simulink model "AR4_robotv5"  (R2021a)
settings: Solver=VariableStepAuto  StartTime=0.0  StopTime=13.7896  RelTol=1e-3
undefined symbols (not defined in the file or in its folder): B, Levenberg, Marquardt, sigbuilder_block, Spline, X, Y, Z
libraries: sm_lib x612, nesl_utility x123, robotcorelib x28, simulink_extras x19, simulink x17, robotmaniplib x9
(part 1 of 14)
settings Model: PacingRate=0.350000  Creator=sense  LastModifiedBy=sense

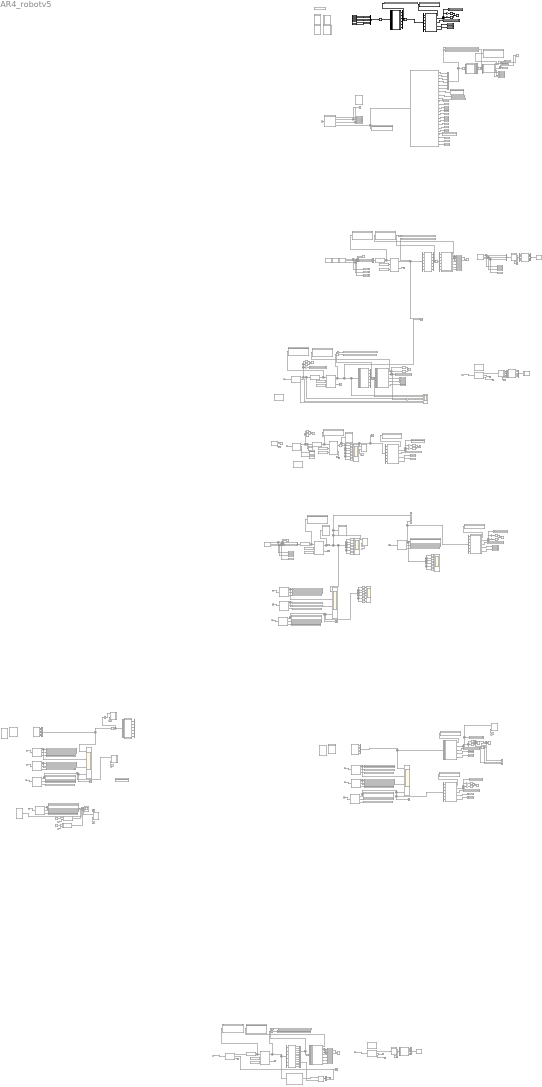
== system AR4_robotv5 ==
  note: task space
  note: joint space
  note: inverse kinematic
  note: Joint angles that achieve the given pose
  note: (Position vector)
  note: Controls importance of position/orientation
  note: Converts the 3D position (translation vector of end-effector) into a 4×4 homogeneous transformation matrix .
  note: Solves the inverse kinematics problem: Given a desired pose (position + orientation), compute the corresponding joint angles.
  note: take the waypoints of the trajectory
      | exert the angles + velocity + acceleration vectors
  note: (velocity vector)
  note: (accel vector)
  note: Joint angles that achieve the given pose
  note: (Position vector)
  note: Controls importance of position/orientation
  note: Converts the 3D position (translation vector of end-effector) into a 4×4 homogeneous transformation matrix .
  note: Solves the inverse kinematics problem: Given a desired pose (position + orientation), compute the corresponding joint angles.
  note: take the waypoints of the trajectory
      | exert the angles + velocity + acceleration vectors
  note: (velocity vector)
  note: (accel vector)
  note: joint space
  note: task space
  note: joint space
  Clock{,1..24} (25 alike) : Clock  Commented=on
  Constant{,2,4..5,8} (5 alike) : Constant  Commented=on  Value=[0 0 0 1 1 1]
  Constant{1,3,6..7,9} (5 alike) : Constant  Commented=on  Value=[0 0 0 0 0 0]
  Constant10 : Constant  Commented=on  Value=[140 60 -60 130 0 120]  VectorParams1D=off
  Constant11 : Constant  Commented=on  Value=[0 30 60 90 120 150 170 140]
  Constant12 : Constant  Commented=on  Value=[0 30 60 90 120 150 170 140]
  Coordinate Transformation Conversion{,1..4} (5 alike) : robotcorelib/Coordinate Transformation Conversion  Commented=on  InputRepresentation=Translation Vector  InputEulerSequence=ZYX  ShowTrVecInputPort=on  OutputRepresentation=Homogeneous Transformation  OutputEulerSequence=ZYX  ShowTrVecOutputPort=on  SimulateUsing=Interpreted execution
      settings: SourceProductBaseCode=NV,RO,RR,UV
  Degrees to Radians : simulink_extras/Transformations/Degrees to Radians  Commented=on
  Degrees to Radians1 : simulink_extras/Transformations/Degrees to Radians
  Degrees to Radians2 : simulink_extras/Transformations/Degrees to Radians  Commented=on
  Demux{,1..12,14,17..18} (16 alike) : Demux  Commented=on  Outputs=6
  Demux13 : Demux  Commented=on  Outputs=2
  Demux15 : Demux  Outputs=6
  Demux16 : Demux  Outputs=6
  Display{,1..76,82..83,85..109,191,263,267,302..304,306..307,309..323,331..332,360} (130 alike) : Display  Commented=on
      Display100 settings: Format=bank
      Display101 settings: Format=bank
      Display102 settings: Format=bank
      Display103 settings: Format=bank
      Display104 settings: Format=bank
      Display105 settings: Format=bank
      Display107 settings: Format=bank
      Display108 settings: Format=bank
      Display109 settings: Format=bank
      Display11 settings: Format=bank
      Display13 settings: Format=bank
      Display18 settings: Format=bank
      Display20 settings: Format=bank
      Display21 settings: Format=bank
      Display22 settings: Format=bank
      Display23 settings: Format=bank
      Display26 settings: Format=bank
      Display28 settings: Format=bank
      Display30 settings: Format=bank
      Display309 settings: Format=bank
      Display31 settings: Format=bank
      Display316 settings: Format=bank
      Display32 settings: Format=bank
      Display33 settings: Format=bank
      Display332 settings: Format=bank
      Display34 settings: Format=bank
      Display39 settings: Format=bank
      Display41 settings: Format=bank
      Display42 settings: Format=bank
      Display47 settings: Format=bank
      Display48 settings: Format=bank
      Display49 settings: Format=bank
      Display50 settings: Format=bank
      Display51 settings: Format=bank
      Display52 settings: Format=bank
      Display53 settings: Format=bank
      Display54 settings: Format=bank
      Display55 settings: Format=bank
      Display56 settings: Format=bank
      Display60 settings: Format=bank
      Display63 settings: Format=bank
      Display66 settings: Format=bank
      Display69 settings: Format=bank
      Display74 settings: Format=bank
      Display82 settings: Format=bank
      Display83 settings: Format=bank
      Display87 settings: Format=bank
      Display90 settings: Format=bank
      Display91 settings: Format=bank
      Display92 settings: Format=bank
      Display93 settings: Format=bank
      Display94 settings: Format=bank
      Display95 settings: Format=bank
      Display96 settings: Format=bank
      Display97 settings: Format=bank
      Display98 settings: Format=bank
      Display99 settings: Format=bank
  Display{77..81,84} (6 alike) : Display
      Display79 settings: Format=bank
  FIK13 : MATLAB Function  Commented=on  TreatAsAtomicUnit=on
  From Workspace : FromWorkspace  VariableName=q1
  From Workspace1 : FromWorkspace  VariableName=q2
  From Workspace2 : FromWorkspace  VariableName=q3
  From Workspace3 : FromWorkspace  VariableName=q4
  From Workspace4 : FromWorkspace  VariableName=q5
  From Workspace5 : FromWorkspace  VariableName=q6
  Gain : Gain  Commented=on  Gain=1000
  Gain{1..5,8..9} (7 alike) : Gain  Commented=on  Gain=0.001
  Gain6 : Gain  Gain=0.001
  Gain7 : Gain  Gain=0.001
  Get Jacobian : robotmaniplib/Get Jacobian  Commented=on  RigidBodyTree=robot  EndEffector=link7  SimulateUsing=Interpreted execution
      settings: SourceProductBaseCode=RO
  Inverse Kinematics{,1,3..4} (4 alike) : robotmaniplib/Inverse Kinematics  Commented=on  RigidBodyTree=robot  EndEffector=link7  ShowInfo=on  SolverName=Levenberg-Marquardt  EnforceJointLimits=on  MaxIterations=1500  MaxTime=10  GradientTolerance=1e-3  SolutionTolerance=1e-3  StepTolerance=1e-14  ErrorChangeTolerance=1e-3  UseErrorDamping=on  DampingBias=0.0025  SimulateUsing=Interpreted execution
  Inverse Kinematics2 : robotmaniplib/Inverse Kinematics  Commented=on  RigidBodyTree=robot  EndEffector=link7  ShowInfo=on  SolverName=Levenberg-Marquardt  EnforceJointLimits=on  MaxIterations=1500  MaxTime=10  GradientTolerance=1e-10  SolutionTolerance=1e-10  StepTolerance=1e-10  ErrorChangeTolerance=1e-10  UseErrorDamping=on  DampingBias=0.0025  SimulateUsing=Interpreted execution
  MATLAB Function : MATLAB Function  Commented=on  TreatAsAtomicUnit=on
  MATLAB Function1 : MATLAB Function  Commented=on  TreatAsAtomicUnit=on
  MATLAB Function10 : MATLAB Function  TreatAsAtomicUnit=on
  MATLAB Function11 : MATLAB Function  Commented=on  TreatAsAtomicUnit=on
  MATLAB Function12 : MATLAB Function  Commented=on  TreatAsAtomicUnit=on
  MATLAB Function13 : MATLAB Function  Commented=on  TreatAsAtomicUnit=on
  MATLAB Function14 : MATLAB Function  Commented=on  TreatAsAtomicUnit=on
  MATLAB Function15 : MATLAB Function  Commented=on  TreatAsAtomicUnit=on
  MATLAB Function16 : MATLAB Function  Commented=on  TreatAsAtomicUnit=on
  MATLAB Function17 : MATLAB Function  Commented=on  TreatAsAtomicUnit=on
  MATLAB Function2 : MATLAB Function  Commented=on  TreatAsAtomicUnit=on
  MATLAB Function3 : MATLAB Function  Commented=on  TreatAsAtomicUnit=on
  MATLAB Function4 : MATLAB Function  Commented=on  TreatAsAtomicUnit=on
  MATLAB Function5 : MATLAB Function  Commented=on  TreatAsAtomicUnit=on
  MATLAB Function6 : MATLAB Function  Commented=on  TreatAsAtomicUnit=on
  MATLAB Function7 : MATLAB Function  Commented=on  TreatAsAtomicUnit=on
  MATLAB Function8 : MATLAB Function  Commented=on  TreatAsAtomicUnit=on
  MATLAB Function9 : MATLAB Function  Commented=on  TreatAsAtomicUnit=on
  Matrix Multiply : Product  Commented=on  Multiplication=Matrix(*)
  Mux{,1,3..6,8..10,12,15,18} (12 alike) : Mux  Commented=on  Inputs=6
  Mux11 : Mux  Commented=on  Inputs=3
  Mux13 : Mux  Inputs=6
  Mux14 : Mux  Inputs=6
  Mux2 : Mux  Commented=on  Inputs=3
  Mux7 : Mux  Commented=on  Inputs=3
  Polynomial Trajectory : robotcorelib/Polynomial Trajectory  Commented=on  WaypointSource=Internal  Waypoints=|  TimePoints=[ 1, 2, 3, 4, 5 ]  TimeInterval=[ 1, 5 ]  Method=B-Spline  ParameterSource=Internal  VelocityBoundaryCondition=zeros(3, 5)  AccelerationBoundaryCondition=zeros(3, 5)  SimulateUsing=Interpreted execution
      | [0.3741, 0.5741, 0.5741, 0.3741, 0.3741;
      |  0.0000, 0.0000, 0.2000, 0.2000, 0.0000;
      |  0.4563, 0.4563, 0.4563, 0.4563, 0.4563]
  Polynomial Trajectory1 : robotcorelib/Polynomial Trajectory  Commented=on  WaypointSource=Internal  Waypoints=|  TimePoints=[ 1, 2, 3, 4, 5 ]  TimeInterval=[ 1, 5 ]  Method=B-Spline  ParameterSource=Internal  VelocityBoundaryCondition=zeros(3, 5)  AccelerationBoundaryCondition=zeros(3, 5)  SimulateUsing=Interpreted execution
      | [0.3741, 0.5741, 0.5741, 0.3741, 0.3741;
      |  0.0000, 0.0000, 0.2000, 0.2000, 0.0000;
      |  0.4563, 0.4563, 0.4563, 0.4563, 0.4563]
  Polynomial Trajectory10 : robotcorelib/Polynomial Trajectory  Commented=on  WaypointSource=Internal  Waypoints=thetatra  TimePoints=t  TimeInterval=time  Method=Cubic Polynomial  ParameterSource=Internal  VelocityBoundaryCondition=zeros(6,145)  AccelerationBoundaryCondition=zeros(6, 4);  SimulateUsing=Interpreted execution
  Polynomial Trajectory11 : robotcorelib/Polynomial Trajectory  Commented=on  WaypointSource=Internal  Waypoints=joint_angles_deg  TimePoints=[ 1, 2, 3, 4, 5 ]  TimeInterval=[0 1 2 3 4 5 6 7]  Method=B-Spline  ParameterSource=Internal  VelocityBoundaryCondition=zeros(3, 5)  AccelerationBoundaryCondition=zeros(3, 5)  SimulateUsing=Interpreted execution
  Polynomial Trajectory12 : robotcorelib/Polynomial Trajectory  Commented=on  WaypointSource=Internal  Waypoints=joint_angles_deg  TimePoints=[0 1 2 3 4 5 6 7 ]  TimeInterval=time  Method=Quintic Polynomial  ParameterSource=Internal  VelocityBoundaryCondition=zeros(6,8)  AccelerationBoundaryCondition=zeros(6,8)  SimulateUsing=Interpreted execution
  Polynomial Trajectory13 : robotcorelib/Polynomial Trajectory  Commented=on  WaypointSource=Internal  Waypoints=joint_angles_deg  TimePoints=[0 1 2 3 4 5 6 7]  TimeInterval=time  Method=Cubic Polynomial  ParameterSource=Internal  VelocityBoundaryCondition=zeros(6,8)  AccelerationBoundaryCondition=zeros(6, 4);  SimulateUsing=Interpreted execution
  Polynomial Trajectory14 : robotcorelib/Polynomial Trajectory  Commented=on  WaypointSource=Internal  Waypoints=joint_angles_deg  TimePoints=[ 1, 2, 3, 4, 5 ]  TimeInterval=[0 1 2 3 4 5 6 7]  Method=B-Spline  ParameterSource=Internal  VelocityBoundaryCondition=zeros(3, 5)  AccelerationBoundaryCondition=zeros(3, 5)  SimulateUsing=Interpreted execution
  Polynomial Trajectory15 : robotcorelib/Polynomial Trajectory  Commented=on  WaypointSource=Internal  Waypoints=joint1_angles  TimePoints=[ 1, 2, 3, 4, 5 ]  TimeInterval=[0 1 2 3 4 5 6 7]  Method=B-Spline  ParameterSource=Internal  VelocityBoundaryCondition=zeros(3, 5)  AccelerationBoundaryCondition=zeros(3, 5)  SimulateUsing=Interpreted execution
  Polynomial Trajectory2 : robotcorelib/Polynomial Trajectory  Commented=on  WaypointSource=Internal  Waypoints=|  TimePoints=[ 2, 4, 6, 8, 10 ]  TimeInterval=[ 1, 20 ]  Method=Quintic Polynomial  ParameterSource=Internal  VelocityBoundaryCondition=zeros(3, 5)  AccelerationBoundaryCondition=zeros(3, 5)  SimulateUsing=Interpreted execution
      | [0.3741, 0.5741, 0.5741, 0.3741, 0.3741;
      |  0.0000, 0.0000, 0.2000, 0.2000, 0.0000;
      |  0.4563, 0.4563, 0.4563, 0.4563, 0.4563]
  Polynomial Trajectory3 : robotcorelib/Polynomial Trajectory  Commented=on  WaypointSource=Internal  Waypoints=|  TimePoints=[ 2, 4, 6, 8, 10 ]  TimeInterval=[ 1, 20 ]  Method=Quintic Polynomial  ParameterSource=Internal  VelocityBoundaryCondition=zeros(3, 5)  AccelerationBoundaryCondition=zeros(3, 5)  SimulateUsing=Interpreted execution
      | [0.3741, 0.5741, 0.5741, 0.3741, 0.3741;
      |  0.0000, 0.0000, 0.2000, 0.2000, 0.0000;
      |  0.4563, 0.4563, 0.4563, 0.4563, 0.4563]
  Polynomial Trajectory4 : robotcorelib/Polynomial Trajectory  Commented=on  WaypointSource=Internal  Waypoints=joint_angles_deg  TimePoints=[ 1, 2, 3, 4, 5 ]  TimeInterval=[0 1 2 3 4 5 6 7]  Method=B-Spline  ParameterSource=Internal  VelocityBoundaryCondition=zeros(3, 5)  AccelerationBoundaryCondition=zeros(3, 5)  SimulateUsing=Interpreted execution
  Polynomial Trajectory5 : robotcorelib/Polynomial Trajectory  Commented=on  WaypointSource=Internal  Waypoints=joint_angles_deg  TimePoints=[0 1 2 3 4 5 6 7 ]  TimeInterval=time  Method=Quintic Polynomial  ParameterSource=Internal  VelocityBoundaryCondition=zeros(6,8)  AccelerationBoundaryCondition=zeros(6,8)  SimulateUsing=Interpreted execution
  Polynomial Trajectory6 : robotcorelib/Polynomial Trajectory  Commented=on  WaypointSource=Internal  Waypoints=joint_angles_deg  TimePoints=[0 1 2 3 4 5 6 7]  TimeInterval=time  Method=Cubic Polynomial  ParameterSource=Internal  VelocityBoundaryCondition=zeros(6,8)  AccelerationBoundaryCondition=zeros(6, 4);  SimulateUsing=Interpreted execution
  Polynomial Trajectory7 : robotcorelib/Polynomial Trajectory  Commented=on  WaypointSource=Internal  Waypoints=thetatra  TimePoints=t  TimeInterval=t  Method=B-Spline  ParameterSource=Internal  VelocityBoundaryCondition=zeros(3, 5)  AccelerationBoundaryCondition=zeros(3, 5)  SimulateUsing=Interpreted execution
  Polynomial Trajectory8 : robotcorelib/Polynomial Trajectory  Commented=on  WaypointSource=Internal  Waypoints=thetatra  TimePoints=[ 1, 2, 3, 4, 5 ]  TimeInterval=t  Method=B-Spline  ParameterSource=Internal  VelocityBoundaryCondition=zeros(3, 5)  AccelerationBoundaryCondition=zeros(3, 5)  SimulateUsing=Interpreted execution
  Polynomial Trajectory9 : robotcorelib/Polynomial Trajectory  Commented=on  WaypointSource=Internal  Waypoints=thetatra  TimePoints=t  TimeInterval=time  Method=Quintic Polynomial  ParameterSource=Internal  VelocityBoundaryCondition=zeros(6,145)  AccelerationBoundaryCondition=zeros(6,145)  SimulateUsing=Interpreted execution
  Radians to Degrees{,1..9,11..12} (12 alike) : simulink_extras/Transformations/Radians to Degrees  Commented=on
  Radians to Degrees10 : simulink_extras/Transformations/Radians to Degrees
  Scope : Scope  Commented=on  NumInputPorts=2
  Scope{1..2,6,9,12} (5 alike) : Scope  Commented=on  NumInputPorts=6
  Scope{5,10,14..15} (4 alike) : Scope  Commented=on  NumInputPorts=4
  Scope{7..8,11,16..17} (5 alike) : Scope  Commented=on
  Scope13 : Scope  Commented=on  NumInputPorts=3
  Scope3 : Scope  Commented=on  NumInputPorts=2
  Scope4 : Scope  Commented=on  NumInputPorts=2
  Selector{,2,16,18,26,28,30} (7 alike) : Selector  Commented=on  InputPortWidth=3  IndexOptions=Index vector (dialog)  Indices=1  OutputSizes=1
  Selector{1,3,17,19,27,29,31} (7 alike) : Selector  Commented=on  InputPortWidth=3  IndexOptions=Index vector (dialog)  Indices=2  OutputSizes=1
  Selector{4,10,20,32} (4 alike) : Selector  Commented=on  InputPortWidth=6  IndexOptions=Index vector (dialog)  Indices=1  OutputSizes=1
  Selector{5,11,21,33} (4 alike) : Selector  Commented=on  InputPortWidth=6  IndexOptions=Index vector (dialog)  Indices=2  OutputSizes=1
  Selector{6,12,22,34} (4 alike) : Selector  Commented=on  InputPortWidth=6  IndexOptions=Index vector (dialog)  Indices=3  OutputSizes=1
  Selector{7,13,23,35} (4 alike) : Selector  Commented=on  InputPortWidth=6  IndexOptions=Index vector (dialog)  Indices=4  OutputSizes=1
  Selector{8,14,24,36} (4 alike) : Selector  Commented=on  InputPortWidth=6  IndexOptions=Index vector (dialog)  Indices=5  OutputSizes=1
  Selector{9,15,25,37} (4 alike) : Selector  Commented=on  InputPortWidth=6  IndexOptions=Index vector (dialog)  Indices=6  OutputSizes=1
  Selector38 : Selector  Commented=on  InputPortWidth=3  IndexOptions=Index vector (dialog)  Indices=3  OutputSizes=1
  Selector39 : Selector  InputPortWidth=3  IndexOptions=Index vector (dialog)  Indices=1  OutputSizes=1
  Selector40 : Selector  InputPortWidth=3  IndexOptions=Index vector (dialog)  Indices=2  OutputSizes=1
  Signal Builder : Subsystem  Tag=STV Subsys  Commented=on  LoadFcn=sigbuilder_block('load');  StartFcn=sigbuilder_block('start');  StopFcn=sigbuilder_block('stop');  ClipboardFcn=sigbuilder_block('clipboard');  mask(Sigbuilder block){tuvar=[0:10]}
      mask help: Simulink:masks:SigbuilderBlock_MD
      mask init:
      | if ~strcmp(get_param(bdroot(gcbh),'SimulationStatus'),'stopped') tuvar = sigbuilder_block('maskInit'); end
      settings: CopyFcn=sigbuilder_block('copy');  DeleteFcn=sigbuilder_block('delete');  ModelCloseFcn=sigbuilder_block('modelClose');  PreSaveFcn=sigbuilder_block('preSave');  PauseFcn=sigbuilder_block('pause');  ContinueFcn=sigbuilder_block('continue');  NameChangeFcn=sigbuilder_block('namechange');  OpenFcn=sigbuilder_block('open',[243 60.75 544.5 355.5 ]);  CloseFcn=sigbuilder_block('close');
      mask Display: plot(0, 0, 100, 100,[2, 2, 32, 32, 2], [68, 8, 8, 68, 68],[32, 2], [38, 38], [32, 19, 2],[53, 60, 44], [32, 17, 17, 2],[16, 16, 31, 31]);txt = getActiveGroup(gcbh);text(2, 100, txt,'verticalAlignment', 'top');
  Signal Builder1 : Subsystem  Tag=STV Subsys  Commented=on  LoadFcn=sigbuilder_block('load');  StartFcn=sigbuilder_block('start');  StopFcn=sigbuilder_block('stop');  ClipboardFcn=sigbuilder_block('clipboard');  mask(Sigbuilder block){tuvar=[0:10]}
      mask help: Simulink:masks:SigbuilderBlock_MD
      mask init:
      | if ~strcmp(get_param(bdroot(gcbh),'SimulationStatus'),'stopped') tuvar = sigbuilder_block('maskInit'); end
      settings: CopyFcn=sigbuilder_block('copy');  DeleteFcn=sigbuilder_block('delete');  ModelCloseFcn=sigbuilder_block('modelClose');  PreSaveFcn=sigbuilder_block('preSave');  PauseFcn=sigbuilder_block('pause');  ContinueFcn=sigbuilder_block('continue');  NameChangeFcn=sigbuilder_block('namechange');  OpenFcn=sigbuilder_block('open',[147.75 66 544.5 355.5 ]);  CloseFcn=sigbuilder_block('close');
      mask Display: plot(0, 0, 100, 100,[2, 2, 32, 32, 2], [68, 8, 8, 68, 68],[32, 2], [38, 38], [32, 19, 2],[53, 60, 44], [32, 17, 17, 2],[16, 16, 31, 31]);txt = getActiveGroup(gcbh);text(2, 100, txt,'verticalAlignment', 'top');
  Signal Builder10 : Subsystem  Tag=STV Subsys  Commented=on  LoadFcn=sigbuilder_block('load');  StartFcn=sigbuilder_block('start');  StopFcn=sigbuilder_block('stop');  ClipboardFcn=sigbuilder_block('clipboard');  mask(Sigbuilder block){tuvar=[0:10]}
      mask help: Simulink:masks:SigbuilderBlock_MD
      mask init:
      | if ~strcmp(get_param(bdroot(gcbh),'SimulationStatus'),'stopped') tuvar = sigbuilder_block('maskInit'); end
      settings: CopyFcn=sigbuilder_block('copy');  DeleteFcn=sigbuilder_block('delete');  ModelCloseFcn=sigbuilder_block('modelClose');  PreSaveFcn=sigbuilder_block('preSave');  PauseFcn=sigbuilder_block('pause');  ContinueFcn=sigbuilder_block('continue');  NameChangeFcn=sigbuilder_block('namechange');  OpenFcn=sigbuilder_block('open',[424.5 118.5 550.5 359.25 ]);  CloseFcn=sigbuilder_block('close');
      mask Display: plot(0, 0, 100, 100,[2, 2, 32, 32, 2], [68, 8, 8, 68, 68],[32, 2], [38, 38], [32, 19, 2],[53, 60, 44], [32, 17, 17, 2],[16, 16, 31, 31]);txt = getActiveGroup(gcbh);text(2, 100, txt,'verticalAlignment', 'top');
  Signal Builder11 : Subsystem  Tag=STV Subsys  Commented=on  LoadFcn=sigbuilder_block('load');  StartFcn=sigbuilder_block('start');  StopFcn=sigbuilder_block('stop');  ClipboardFcn=sigbuilder_block('clipboard');  mask(Sigbuilder block){tuvar=[0:10]}
      mask help: Simulink:masks:SigbuilderBlock_MD
      mask init:
      | if ~strcmp(get_param(bdroot(gcbh),'SimulationStatus'),'stopped') tuvar = sigbuilder_block('maskInit'); end
      settings: CopyFcn=sigbuilder_block('copy');  DeleteFcn=sigbuilder_block('delete');  ModelCloseFcn=sigbuilder_block('modelClose');  PreSaveFcn=sigbuilder_block('preSave');  PauseFcn=sigbuilder_block('pause');  ContinueFcn=sigbuilder_block('continue');  NameChangeFcn=sigbuilder_block('namechange');  OpenFcn=sigbuilder_block('open',[424.5 118.5 550.5 359.25 ]);  CloseFcn=sigbuilder_block('close');
      mask Display: plot(0, 0, 100, 100,[2, 2, 32, 32, 2], [68, 8, 8, 68, 68],[32, 2], [38, 38], [32, 19, 2],[53, 60, 44], [32, 17, 17, 2],[16, 16, 31, 31]);txt = getActiveGroup(gcbh);text(2, 100, txt,'verticalAlignment', 'top');
  Signal Builder12 : Subsystem  Tag=STV Subsys  Commented=on  LoadFcn=sigbuilder_block('load');  StartFcn=sigbuilder_block('start');  StopFcn=sigbuilder_block('stop');  ClipboardFcn=sigbuilder_block('clipboard');  mask(Sigbuilder block){tuvar=[0:10]}
      mask help: Simulink:masks:SigbuilderBlock_MD
      mask init:
      | if ~strcmp(get_param(bdroot(gcbh),'SimulationStatus'),'stopped') tuvar = sigbuilder_block('maskInit'); end
      settings: CopyFcn=sigbuilder_block('copy');  DeleteFcn=sigbuilder_block('delete');  ModelCloseFcn=sigbuilder_block('modelClose');  PreSaveFcn=sigbuilder_block('preSave');  PauseFcn=sigbuilder_block('pause');  ContinueFcn=sigbuilder_block('continue');  NameChangeFcn=sigbuilder_block('namechange');  OpenFcn=sigbuilder_block('open',[424.5 118.5 550.5 359.25 ]);  CloseFcn=sigbuilder_block('close');
      mask Display: plot(0, 0, 100, 100,[2, 2, 32, 32, 2], [68, 8, 8, 68, 68],[32, 2], [38, 38], [32, 19, 2],[53, 60, 44], [32, 17, 17, 2],[16, 16, 31, 31]);txt = getActiveGroup(gcbh);text(2, 100, txt,'verticalAlignment', 'top');
  Signal Builder13 : Subsystem  Tag=STV Subsys  Commented=on  LoadFcn=sigbuilder_block('load');  StartFcn=sigbuilder_block('start');  StopFcn=sigbuilder_block('stop');  ClipboardFcn=sigbuilder_block('clipboard');  mask(Sigbuilder block){tuvar=[0:10]}
      mask help: Simulink:masks:SigbuilderBlock_MD
      mask init:
      | if ~strcmp(get_param(bdroot(gcbh),'SimulationStatus'),'stopped') tuvar = sigbuilder_block('maskInit'); end
      settings: CopyFcn=sigbuilder_block('copy');  DeleteFcn=sigbuilder_block('delete');  ModelCloseFcn=sigbuilder_block('modelClose');  PreSaveFcn=sigbuilder_block('preSave');  PauseFcn=sigbuilder_block('pause');  ContinueFcn=sigbuilder_block('continue');  NameChangeFcn=sigbuilder_block('namechange');  OpenFcn=sigbuilder_block('open',[437.6 153 550.4 359.25 ]);  CloseFcn=sigbuilder_block('close');
      mask Display: plot(0, 0, 100, 100,[2, 2, 32, 32, 2], [68, 8, 8, 68, 68],[32, 2], [38, 38], [32, 19, 2],[53, 60, 44], [32, 17, 17, 2],[16, 16, 31, 31]);txt = getActiveGroup(gcbh);text(2, 100, txt,'verticalAlignment', 'top');
  Signal Builder14 : Subsystem  Tag=STV Subsys  Commented=on  LoadFcn=sigbuilder_block('load');  StartFcn=sigbuilder_block('start');  StopFcn=sigbuilder_block('stop');  ClipboardFcn=sigbuilder_block('clipboard');  mask(Sigbuilder block){tuvar=[0:10]}
      mask help: Simulink:masks:SigbuilderBlock_MD
      mask init:
      | if ~strcmp(get_param(bdroot(gcbh),'SimulationStatus'),'stopped') tuvar = sigbuilder_block('maskInit'); end
      settings: CopyFcn=sigbuilder_block('copy');  DeleteFcn=sigbuilder_block('delete');  ModelCloseFcn=sigbuilder_block('modelClose');  PreSaveFcn=sigbuilder_block('preSave');  PauseFcn=sigbuilder_block('pause');  ContinueFcn=sigbuilder_block('continue');  NameChangeFcn=sigbuilder_block('namechange');  OpenFcn=sigbuilder_block('open',[255.75 82.5 544.5 355.5 ]);  CloseFcn=sigbuilder_block('close');
      mask Display: plot(0, 0, 100, 100,[2, 2, 32, 32, 2], [68, 8, 8, 68, 68],[32, 2], [38, 38], [32, 19, 2],[53, 60, 44], [32, 17, 17, 2],[16, 16, 31, 31]);txt = getActiveGroup(gcbh);text(2, 100, txt,'verticalAlignment', 'top');
  Signal Builder15 : Subsystem  Tag=STV Subsys  Commented=on  LoadFcn=sigbuilder_block('load');  StartFcn=sigbuilder_block('start');  StopFcn=sigbuilder_block('stop');  ClipboardFcn=sigbuilder_block('clipboard');  mask(Sigbuilder block){tuvar=[0:10]}
      mask help: Simulink:masks:SigbuilderBlock_MD
      mask init:
      | if ~strcmp(get_param(bdroot(gcbh),'SimulationStatus'),'stopped') tuvar = sigbuilder_block('maskInit'); end
      settings: CopyFcn=sigbuilder_block('copy');  DeleteFcn=sigbuilder_block('delete');  ModelCloseFcn=sigbuilder_block('modelClose');  PreSaveFcn=sigbuilder_block('preSave');  PauseFcn=sigbuilder_block('pause');  ContinueFcn=sigbuilder_block('continue');  NameChangeFcn=sigbuilder_block('namechange');  OpenFcn=sigbuilder_block('open',[424.5 118.5 550.5 359.25 ]);  CloseFcn=sigbuilder_block('close');
      mask Display: plot(0, 0, 100, 100,[2, 2, 32, 32, 2], [68, 8, 8, 68, 68],[32, 2], [38, 38], [32, 19, 2],[53, 60, 44], [32, 17, 17, 2],[16, 16, 31, 31]);txt = getActiveGroup(gcbh);text(2, 100, txt,'verticalAlignment', 'top');
  Signal Builder2 : Subsystem  Tag=STV Subsys  Commented=on  LoadFcn=sigbuilder_block('load');  StartFcn=sigbuilder_block('start');  StopFcn=sigbuilder_block('stop');  ClipboardFcn=sigbuilder_block('clipboard');  mask(Sigbuilder block){tuvar=[0:10]}
      mask help: Simulink:masks:SigbuilderBlock_MD
      mask init:
      | if ~strcmp(get_param(bdroot(gcbh),'SimulationStatus'),'stopped') tuvar = sigbuilder_block('maskInit'); end
      settings: CopyFcn=sigbuilder_block('copy');  DeleteFcn=sigbuilder_block('delete');  ModelCloseFcn=sigbuilder_block('modelClose');  PreSaveFcn=sigbuilder_block('preSave');  PauseFcn=sigbuilder_block('pause');  ContinueFcn=sigbuilder_block('continue');  NameChangeFcn=sigbuilder_block('namechange');  OpenFcn=sigbuilder_block('open',[255.75 82.5 544.5 355.5 ]);  CloseFcn=sigbuilder_block('close');
      mask Display: plot(0, 0, 100, 100,[2, 2, 32, 32, 2], [68, 8, 8, 68, 68],[32, 2], [38, 38], [32, 19, 2],[53, 60, 44], [32, 17, 17, 2],[16, 16, 31, 31]);txt = getActiveGroup(gcbh);text(2, 100, txt,'verticalAlignment', 'top');
  Signal Builder3 : Subsystem  Tag=STV Subsys  Commented=on  LoadFcn=sigbuilder_block('load');  StartFcn=sigbuilder_block('start');  StopFcn=sigbuilder_block('stop');  ClipboardFcn=sigbuilder_block('clipboard');  mask(Sigbuilder block){tuvar=[0:10]}
      mask help: Simulink:masks:SigbuilderBlock_MD
      mask init:
      | if ~strcmp(get_param(bdroot(gcbh),'SimulationStatus'),'stopped') tuvar = sigbuilder_block('maskInit'); end
      settings: CopyFcn=sigbuilder_block('copy');  DeleteFcn=sigbuilder_block('delete');  ModelCloseFcn=sigbuilder_block('modelClose');  PreSaveFcn=sigbuilder_block('preSave');  PauseFcn=sigbuilder_block('pause');  ContinueFcn=sigbuilder_block('continue');  NameChangeFcn=sigbuilder_block('namechange');  OpenFcn=sigbuilder_block('open',[252 18.75 544.5 355.5 ]);  CloseFcn=sigbuilder_block('close');
      mask Display: plot(0, 0, 100, 100,[2, 2, 32, 32, 2], [68, 8, 8, 68, 68],[32, 2], [38, 38], [32, 19, 2],[53, 60, 44], [32, 17, 17, 2],[16, 16, 31, 31]);txt = getActiveGroup(gcbh);text(2, 100, txt,'verticalAlignment', 'top');
  Signal Builder4 : Subsystem  Tag=STV Subsys  Commented=on  LoadFcn=sigbuilder_block('load');  StartFcn=sigbuilder_block('start');  StopFcn=sigbuilder_block('stop');  ClipboardFcn=sigbuilder_block('clipboard');  mask(Sigbuilder block){tuvar=[0:10]}
      mask help: Simulink:masks:SigbuilderBlock_MD
      mask init:
      | if ~strcmp(get_param(bdroot(gcbh),'SimulationStatus'),'stopped') tuvar = sigbuilder_block('maskInit'); end
      settings: CopyFcn=sigbuilder_block('copy');  DeleteFcn=sigbuilder_block('delete');  ModelCloseFcn=sigbuilder_block('modelClose');  PreSaveFcn=sigbuilder_block('preSave');  PauseFcn=sigbuilder_block('pause');  ContinueFcn=sigbuilder_block('continue');  NameChangeFcn=sigbuilder_block('namechange');  OpenFcn=sigbuilder_block('open',[252 18.75 544.5 355.5 ]);  CloseFcn=sigbuilder_block('close');
      mask Display: plot(0, 0, 100, 100,[2, 2, 32, 32, 2], [68, 8, 8, 68, 68],[32, 2], [38, 38], [32, 19, 2],[53, 60, 44], [32, 17, 17, 2],[16, 16, 31, 31]);txt = getActiveGroup(gcbh);text(2, 100, txt,'verticalAlignment', 'top');
  Signal Builder5 : Subsystem  Tag=STV Subsys  Commented=on  LoadFcn=sigbuilder_block('load');  StartFcn=sigbuilder_block('start');  StopFcn=sigbuilder_block('stop');  ClipboardFcn=sigbuilder_block('clipboard');  mask(Sigbuilder block){tuvar=[0:10]}
      mask help: Simulink:masks:SigbuilderBlock_MD
      mask init:
      | if ~strcmp(get_param(bdroot(gcbh),'SimulationStatus'),'stopped') tuvar = sigbuilder_block('maskInit'); end
      settings: CopyFcn=sigbuilder_block('copy');  DeleteFcn=sigbuilder_block('delete');  ModelCloseFcn=sigbuilder_block('modelClose');  PreSaveFcn=sigbuilder_block('preSave');  PauseFcn=sigbuilder_block('pause');  ContinueFcn=sigbuilder_block('continue');  NameChangeFcn=sigbuilder_block('namechange');  OpenFcn=sigbuilder_block('open',[424.5 118.5 550.5 359.25 ]);  CloseFcn=sigbuilder_block('close');
      mask Display: plot(0, 0, 100, 100,[2, 2, 32, 32, 2], [68, 8, 8, 68, 68],[32, 2], [38, 38], [32, 19, 2],[53, 60, 44], [32, 17, 17, 2],[16, 16, 31, 31]);txt = getActiveGroup(gcbh);text(2, 100, txt,'verticalAlignment', 'top');
  Signal Builder6 : Subsystem  Tag=STV Subsys  Commented=on  LoadFcn=sigbuilder_block('load');  StartFcn=sigbuilder_block('start');  StopFcn=sigbuilder_block('stop');  ClipboardFcn=sigbuilder_block('clipboard');  mask(Sigbuilder block){tuvar=[0:10]}
      mask help: Simulink:masks:SigbuilderBlock_MD
      mask init:
      | if ~strcmp(get_param(bdroot(gcbh),'SimulationStatus'),'stopped') tuvar = sigbuilder_block('maskInit'); end
      settings: CopyFcn=sigbuilder_block('copy');  DeleteFcn=sigbuilder_block('delete');  ModelCloseFcn=sigbuilder_block('modelClose');  PreSaveFcn=sigbuilder_block('preSave');  PauseFcn=sigbuilder_block('pause');  ContinueFcn=sigbuilder_block('continue');  NameChangeFcn=sigbuilder_block('namechange');  OpenFcn=sigbuilder_block('open',[424.5 118.5 550.5 359.25 ]);  CloseFcn=sigbuilder_block('close');
      mask Display: plot(0, 0, 100, 100,[2, 2, 32, 32, 2], [68, 8, 8, 68, 68],[32, 2], [38, 38], [32, 19, 2],[53, 60, 44], [32, 17, 17, 2],[16, 16, 31, 31]);txt = getActiveGroup(gcbh);text(2, 100, txt,'verticalAlignment', 'top');
  Signal Builder7 : Subsystem  Tag=STV Subsys  Commented=on  LoadFcn=sigbuilder_block('load');  StartFcn=sigbuilder_block('start');  StopFcn=sigbuilder_block('stop');  ClipboardFcn=sigbuilder_block('clipboard');  mask(Sigbuilder block){tuvar=[0:10]}
      mask help: Simulink:masks:SigbuilderBlock_MD
      mask init:
      | if ~strcmp(get_param(bdroot(gcbh),'SimulationStatus'),'stopped') tuvar = sigbuilder_block('maskInit'); end
      settings: CopyFcn=sigbuilder_block('copy');  DeleteFcn=sigbuilder_block('delete');  ModelCloseFcn=sigbuilder_block('modelClose');  PreSaveFcn=sigbuilder_block('preSave');  PauseFcn=sigbuilder_block('pause');  ContinueFcn=sigbuilder_block('continue');  NameChangeFcn=sigbuilder_block('namechange');  OpenFcn=sigbuilder_block('open',[464.25 150.75 550.5 359.25 ]);  CloseFcn=sigbuilder_block('close');
      mask Display: plot(0, 0, 100, 100,[2, 2, 32, 32, 2], [68, 8, 8, 68, 68],[32, 2], [38, 38], [32, 19, 2],[53, 60, 44], [32, 17, 17, 2],[16, 16, 31, 31]);txt = getActiveGroup(gcbh);text(2, 100, txt,'verticalAlignment', 'top');
  Signal Builder8 : Subsystem  Tag=STV Subsys  Commented=on  LoadFcn=sigbuilder_block('load');  StartFcn=sigbuilder_block('start');  StopFcn=sigbuilder_block('stop');  ClipboardFcn=sigbuilder_block('clipboard');  mask(Sigbuilder block){tuvar=[0:10]}
      mask help: Simulink:masks:SigbuilderBlock_MD
      mask init:
      | if ~strcmp(get_param(bdroot(gcbh),'SimulationStatus'),'stopped') tuvar = sigbuilder_block('maskInit'); end
      settings: CopyFcn=sigbuilder_block('copy');  DeleteFcn=sigbuilder_block('delete');  ModelCloseFcn=sigbuilder_block('modelClose');  PreSaveFcn=sigbuilder_block('preSave');  PauseFcn=sigbuilder_block('pause');  ContinueFcn=sigbuilder_block('continue');  NameChangeFcn=sigbuilder_block('namechange');  OpenFcn=sigbuilder_block('open',[424.5 118.5 550.5 359.25 ]);  CloseFcn=sigbuilder_block('close');
      mask Display: plot(0, 0, 100, 100,[2, 2, 32, 32, 2], [68, 8, 8, 68, 68],[32, 2], [38, 38], [32, 19, 2],[53, 60, 44], [32, 17, 17, 2],[16, 16, 31, 31]);txt = getActiveGroup(gcbh);text(2, 100, txt,'verticalAlignment', 'top');
  Signal Builder9 : Subsystem  Tag=STV Subsys  Commented=on  LoadFcn=sigbuilder_block('load');  StartFcn=sigbuilder_block('start');  StopFcn=sigbuilder_block('stop');  ClipboardFcn=sigbuilder_block('clipboard');  mask(Sigbuilder block){tuvar=[0:10]}
      mask help: Simulink:masks:SigbuilderBlock_MD
      mask init:
      | if ~strcmp(get_param(bdroot(gcbh),'SimulationStatus'),'stopped') tuvar = sigbuilder_block('maskInit'); end
      settings: CopyFcn=sigbuilder_block('copy');  DeleteFcn=sigbuilder_block('delete');  ModelCloseFcn=sigbuilder_block('modelClose');  PreSaveFcn=sigbuilder_block('preSave');  PauseFcn=sigbuilder_block('pause');  ContinueFcn=sigbuilder_block('continue');  NameChangeFcn=sigbuilder_block('namechange');  OpenFcn=sigbuilder_block('open',[437.6 153 550.4 359.25 ]);  CloseFcn=sigbuilder_block('close');
      mask Display: plot(0, 0, 100, 100,[2, 2, 32, 32, 2], [68, 8, 8, 68, 68],[32, 2], [38, 38], [32, 19, 2],[53, 60, 44], [32, 17, 17, 2],[16, 16, 31, 31]);txt = getActiveGroup(gcbh);text(2, 100, txt,'verticalAlignment', 'top');
  Subsystem : Subsystem
  Subsystem1 : Subsystem  Commented=on
  Subsystem10 : Subsystem  Commented=on
  Subsystem11 : Subsystem  Commented=on
  Subsystem12 : Subsystem  Commented=on
  Subsystem13 : Subsystem  Commented=on
  Subsystem14 : Subsystem  Commented=on
  Subsystem2 : Subsystem  Commented=on
  Subsystem3 : Subsystem  Commented=on
  Subsystem4 : Subsystem  Commented=on
  Subsystem5 : Subsystem  Commented=on
  Subsystem6 : Subsystem  Commented=on
  Subsystem7 : Subsystem  Commented=on
  Subsystem8 : Subsystem  Commented=on
  Subsystem9 : Subsystem  Commented=on
  Terminator{,1..14} (15 alike) : Terminator  Commented=on
  Trapezoidal Velocity Profile Trajectory : robotcorelib/Trapezoidal Velocity Profile Trajectory  Commented=on  WaypointSource=Internal  Waypoints=|  NumParams=0  Parameter1=Peak Velocity  Parameter2=End Time  ParameterSource=Internal  PeakVelocity=[ 2; 2 ]  Acceleration=[ 1; 2 ]  EndTime=[ 1; 1 ]  AccelTime=[ 1; 2 ]  SimulateUsing=Interpreted execution
      | [0.3741, 0.5741, 0.5741, 0.3741, 0.3741;
      |  0.0000, 0.0000, 0.2000, 0.2000, 0.0000;
      |  0.4563, 0.4563, 0.4563, 0.4563, 0.4563]
      settings: SourceProductBaseCode=NV,RO,RR,UV
  Trapezoidal Velocity Profile Trajectory1 : robotcorelib/Trapezoidal Velocity Profile Trajectory  Commented=on  WaypointSource=Internal  Waypoints=|  NumParams=0  Parameter1=Peak Velocity  Parameter2=End Time  ParameterSource=Internal  PeakVelocity=[ 2; 2 ]  Acceleration=[ 1; 2 ]  EndTime=[ 1; 1 ]  AccelTime=[ 1; 2 ]  SimulateUsing=Interpreted execution
      | [0.3741, 0.5741, 0.5741, 0.3741, 0.3741;
      |  0.0000, 0.0000, 0.2000, 0.2000, 0.0000;
      |  0.4563, 0.4563, 0.4563, 0.4563, 0.4563]
      settings: SourceProductBaseCode=NV,RO,RR,UV
  Trapezoidal Velocity Profile Trajectory2 : robotcorelib/Trapezoidal Velocity Profile Trajectory  Commented=on  WaypointSource=Internal  Waypoints=|  NumParams=0  Parameter1=Peak Velocity  Parameter2=End Time  ParameterSource=Internal  PeakVelocity=[ 2; 2 ]  Acceleration=[ 1; 2 ]  EndTime=[ 1; 1 ]  AccelTime=[ 1; 2 ]  SimulateUsing=Interpreted execution
      | [0.3741, 0.5741, 0.5741, 0.3741, 0.3741;
      |  0.0000, 0.0000, 0.2000, 0.2000, 0.0000;
      |  0.4563, 0.4563, 0.4563, 0.4563, 0.4563]
      settings: SourceProductBaseCode=NV,RO,RR,UV
  Trapezoidal Velocity Profile Trajectory3 : robotcorelib/Trapezoidal Velocity Profile Trajectory  Commented=on  WaypointSource=Internal  Waypoints=|  NumParams=0  Parameter1=Peak Velocity  Parameter2=End Time  ParameterSource=Internal  PeakVelocity=[ 2; 2 ]  Acceleration=[ 1; 2 ]  EndTime=[ 1; 1 ]  AccelTime=[ 1; 2 ]  SimulateUsing=Interpreted execution
      | [0.3741, 0.5741, 0.5741, 0.3741, 0.3741;
      |  0.0000, 0.0000, 0.2000, 0.2000, 0.0000;
      |  0.4563, 0.4563, 0.4563, 0.4563, 0.4563]
      settings: SourceProductBaseCode=NV,RO,RR,UV
  XD YD{1..3,6} (4 alike) : simulink/Sinks/XY Graph  Commented=on  xmin=-100  xmax=100  ymin=-100  ymax=100  st=-1
  XY Graph : simulink/Sinks/XY Graph  Commented=on  xmin=-1  xmax=1  ymin=-1  ymax=1  st=-1
  XY input : simulink/Sinks/XY Graph  Commented=on  xmin=0.3  xmax=1  ymin=-0.2  ymax=0.6  st=-1
  XY out : simulink/Sinks/XY Graph  Commented=on  xmin=300  xmax=1000  ymin=-200  ymax=600  st=-1
  circle3 : MATLAB Function  Commented=on  TreatAsAtomicUnit=on
  curve : Subsystem  Tag=STV Subsys  Commented=on  LoadFcn=sigbuilder_block('load');  StartFcn=sigbuilder_block('start');  StopFcn=sigbuilder_block('stop');  ClipboardFcn=sigbuilder_block('clipboard');  mask(Sigbuilder block){tuvar=[0:10]}
      mask help: Simulink:masks:SigbuilderBlock_MD
      mask init:
      | if ~strcmp(get_param(bdroot(gcbh),'SimulationStatus'),'stopped') tuvar = sigbuilder_block('maskInit'); end
      settings: CopyFcn=sigbuilder_block('copy');  DeleteFcn=sigbuilder_block('delete');  ModelCloseFcn=sigbuilder_block('modelClose');  PreSaveFcn=sigbuilder_block('preSave');  PauseFcn=sigbuilder_block('pause');  ContinueFcn=sigbuilder_block('continue');  NameChangeFcn=sigbuilder_block('namechange');  OpenFcn=sigbuilder_block('open',[437.6 153 550.4 359.25 ]);  CloseFcn=sigbuilder_block('close');
      mask Display: plot(0, 0, 100, 100,[2, 2, 32, 32, 2], [68, 8, 8, 68, 68],[32, 2], [38, 38], [32, 19, 2],[53, 60, 44], [32, 17, 17, 2],[16, 16, 31, 31]);txt = getActiveGroup(gcbh);text(2, 100, txt,'verticalAlignment', 'top');
  xy  interpolation1 : simulink/Sinks/XY Graph  Commented=on  xmin=0.3  xmax=1  ymin=-0.2  ymax=0.6  st=-1
  xy  interpolation2 : simulink/Sinks/XY Graph  Commented=on  xmin=0.3  xmax=1  ymin=-0.2  ymax=0.6  st=-1
  xy  interpolation3 : simulink/Sinks/XY Graph  Commented=on  xmin=-1000  xmax=1000  ymin=-1000  ymax=1000  st=-1
  xy  interpolation4 : simulink/Sinks/XY Graph  Commented=on  xmin=0.3  xmax=1  ymin=-0.2  ymax=0.6  st=-1
  xy  interpolation5 : simulink/Sinks/XY Graph  Commented=on  xmin=-1000  xmax=1000  ymin=-1000  ymax=1000  st=-1
  xy  interpolation6 : simulink/Sinks/XY Graph  xmin=0.3  xmax=1  ymin=-0.2  ymax=0.6  st=-1
  xy with interpolation : simulink/Sinks/XY Graph  Commented=on  xmin=0.3  xmax=1  ymin=-0.2  ymax=0.6  st=-1
  xy without interpolation1 : simulink/Sinks/XY Graph  Commented=on  xmin=.3  xmax=1  ymin=-.2  ymax=.6  st=-1
  xy without interpolation2 : simulink/Sinks/XY Graph  Commented=on  xmin=.3  xmax=1  ymin=-.2  ymax=.6  st=-1
  wires:
  MATLAB Function2/5(Rx) -> Display25/1
  Demux1/6 -> MATLAB Function5/6(theta6)
  MATLAB Function5/6(Ry) -> Display360/1
  Demux1/5 -> MATLAB Function5/5(theta5)
  Demux1/1 -> MATLAB Function5/1(theta1)
  MATLAB Function5/3(Y) -> XD YD1/1, Display267/1
  Demux1/2 -> MATLAB Function5/2(theta2)
  MATLAB Function5/2(X) -> Display331/1
  MATLAB Function6/6(Ry) -> Display12/1
  MATLAB Function6/1(H) -> Display11/1
  MATLAB Function6/7(Rx) -> Display5/1
  Demux3/3 -> MATLAB Function6/3(theta3)
  Demux3/1 -> MATLAB Function6/1(theta1)
  MATLAB Function6/5(Rz) -> Display7/1
  MATLAB Function6/2(X) -> XD YD2/1, Display10/1
  Demux3/4 -> MATLAB Function6/4(theta4)
  Clock/1 -> Polynomial Trajectory/1
  Demux3/2 -> MATLAB Function6/2(theta2)
  MATLAB Function6/4(Z) -> Display6/1
  Demux3/6 -> MATLAB Function6/6(theta6)
  Demux5/6 -> MATLAB Function2/6(theta6)
  Demux5/2 -> MATLAB Function2/2(theta2)
  Mux7/1 -> Subsystem10/1(In1)
  Demux3/5 -> MATLAB Function6/5(theta5)
  Clock1/1 -> Trapezoidal Velocity Profile Trajectory/1
  Signal Builder1/1(x) -> Display35/1, Mux7/1
  Signal Builder1/2(y) -> Display36/1, Mux7/2
  Subsystem4/6(output5) -> Mux6/6
  Subsystem4/5(output4) -> Mux6/5
  Demux9/4 -> Subsystem4/4(input3)
  Demux9/3 -> Subsystem4/3(input2)
  Demux9/2 -> Subsystem4/2(input1)
  Subsystem4/1(output) -> Mux6/1
  Mux6/1 -> Subsystem9/1(Radians in)
  Demux9/5 -> Subsystem4/5(input4)
  Subsystem5/3(output2) -> Mux5/3
  Subsystem5/1(output) -> Mux5/1
  MATLAB Function5/1(H) -> Display332/1
  Subsystem5/6(output5) -> Mux5/6
  Subsystem5/5(output4) -> Mux5/5
  Subsystem5/2(output1) -> Mux5/2
  Subsystem5/4(output3) -> Mux5/4
  MATLAB Function2/1(H) -> Display18/1
  Demux5/5 -> MATLAB Function2/5(theta5)
  Demux5/4 -> MATLAB Function2/4(theta4)
  MATLAB Function2/3(Rz) -> Display27/1
  Subsystem7/2(Info) -> Terminator4/1
  Subsystem7/1(Config) -> Demux8/1
  MATLAB Function6/3(Y) -> XD YD2/2, Display8/1
  Trapezoidal Velocity Profile Trajectory/3 -> Terminator6/1
  Polynomial Trajectory/3 -> Scope1/6
  Inverse Kinematics/1 -> Scope4/1, Display4/1, Demux2/1
  Constant/1 -> Inverse Kinematics/2
  Mux2/1 -> Coordinate Transformation Conversion/1
  Demux4/6 -> Subsystem3/6(input5)
  Subsystem3/6(output5) -> Mux3/6
  Subsystem3/5(output4) -> Mux3/5
  Subsystem3/2(output1) -> Mux3/2
  Subsystem3/4(output3) -> Mux3/4
  Mux3/1 -> Radians to Degrees2/1, Radians to Degrees4/1
  Demux4/2 -> Subsystem3/2(input1)
  Demux4/5 -> Subsystem3/5(input4)
  Inverse Kinematics1/1 -> Scope4/2, Scope1/1, Demux4/1, Radians to Degrees5/1
  Subsystem3/1(output) -> Mux3/1
  Demux4/4 -> Subsystem3/4(input3)
  Inverse Kinematics/2 -> Terminator/1
  Trapezoidal Velocity Profile Trajectory/2 -> Terminator5/1
  Demux4/1 -> Subsystem3/1(input0)
  Subsystem3/3(output2) -> Mux3/3
  Constant3/1 -> Inverse Kinematics1/3
  Coordinate Transformation Conversion1/1 -> Display20/1, Inverse Kinematics1/1
  Constant2/1 -> Inverse Kinematics1/2
  MATLAB Function2/4(Ry) -> Display19/1
  Demux5/3 -> MATLAB Function2/3(theta3)
  Signal Builder2/3(z) -> Mux2/3, Display15/1
  MATLAB Function5/4(Z) -> XD YD1/2, Display191/1
  Subsystem2/6(output5) -> Mux1/6
  Subsystem2/2(output1) -> Mux1/2
  Subsystem2/4(output3) -> Mux1/4
  Demux2/1 -> Subsystem2/1(input0)
  Subsystem2/1(output) -> Mux1/1
  Demux2/4 -> Subsystem2/4(input3)
  Trapezoidal Velocity Profile Trajectory/1 -> Subsystem7/1(In1)
  Radians to Degrees1/1 -> Demux3/1
  Polynomial Trajectory/2 -> Scope1/5
  Mux1/1 -> Radians to Degrees12/1, Radians to Degrees1/1
  Demux2/2 -> Subsystem2/2(input1)
  Subsystem2/5(output4) -> Mux1/5
  Demux2/3 -> Subsystem2/3(input2)
  Mux5/1 -> Subsystem6/1(Radians in)
  FIK13/14(l3) -> Display314/1
  FIK13/1(theta1) -> Mux18/1
  Subsystem4/4(output3) -> Mux6/4
  Subsystem1/5(output4) -> Mux/5
  Subsystem1/2(output1) -> Mux/2
  Subsystem1/6(output5) -> Mux/6
  Demux1/4 -> MATLAB Function5/4(theta4)
  FIK13/5(theta5) -> Mux18/5
  Demux4/3 -> Subsystem3/3(input2)
  Subsystem10/1(Config) -> Demux9/1
  Demux1/3 -> MATLAB Function5/3(theta3)
  FIK13/13(l2) -> Display313/1
  Subsystem1/4(output3) -> Mux/4
  circle3/4(H) -> Display309/1, FIK13/1(H)
  circle3/3(zd) -> XD YD3/2, Display310/1
  Subsystem4/3(output2) -> Mux6/3
  FIK13/22(RY) -> Display303/1
  FIK13/10(X) -> Display318/1
  Signal Builder1/3(z) -> Display37/1, Mux7/3
  FIK13/18(theta_D) -> Display322/1
  Demux/6 -> Subsystem1/6(input5)
  Subsystem2/3(output2) -> Mux1/3
  FIK13/21(RZ) -> Display302/1
  Demux/5 -> Subsystem1/5(input4)
  FIK13/15(l4) -> Display315/1
  Subsystem1/1(output) -> Mux/1
  circle3/1(xd) -> Display307/1
  circle3/2(yd) -> XD YD3/1, Display311/1
  Mux/1 -> Radians to Degrees/1
  MATLAB Function5/7(Rx) -> Display1/1
  Clock3/1 -> circle3/1(u)
  Degrees to Radians/1 -> Demux/1
  Mux18/1 -> Degrees to Radians/1, Display/1
  Demux/4 -> Subsystem1/4(input3)
  FIK13/9(Oc0) -> Display317/1
  Radians to Degrees/1 -> Display3/1, Demux1/1
  MATLAB Function5/5(Rz) -> Display263/1
  FIK13/19(theta_E) -> Display323/1
  FIK13/3(theta3) -> Mux18/3
  Demux/2 -> Subsystem1/2(input1)
  FIK13/17(theta_C) -> Display321/1
  FIK13/20(R63) -> Display316/1
  Demux2/5 -> Subsystem2/5(input4)
  FIK13/16(theta_B) -> Display320/1
  FIK13/4(theta4) -> Mux18/4
  FIK13/8(O60) -> Display2/1
  Demux9/1 -> Subsystem4/1(input0)
  FIK13/6(theta6) -> Mux18/6
  Demux2/6 -> Subsystem2/6(input5)
  Coordinate Transformation Conversion/1 -> Display13/1, Inverse Kinematics/1
  FIK13/12(l1) -> Display312/1
  Signal Builder2/2(y) -> Display16/1, XY Graph/2, Mux2/2
  Constant1/1 -> Inverse Kinematics/3
  Demux5/1 -> MATLAB Function2/1(theta1)
  Subsystem10/2(Info) -> Terminator7/1
  FIK13/2(theta2) -> Mux18/2
  Subsystem1/3(output2) -> Mux/3
  Demux/1 -> Subsystem1/1(input0)
  Demux/3 -> Subsystem1/3(input2)
  FIK13/7(R60) -> Display306/1
  FIK13/23(RX) -> Display304/1
  Inverse Kinematics1/2 -> Terminator1/1
  FIK13/11(Y) -> Display319/1
  Subsystem4/2(output1) -> Mux6/2
  Demux9/6 -> Subsystem4/6(input5)
  Demux8/1 -> Subsystem5/1(input0)
  Demux8/2 -> Subsystem5/2(input1)
  Demux8/3 -> Subsystem5/3(input2)
  Demux8/4 -> Subsystem5/4(input3)
  Demux8/5 -> Subsystem5/5(input4)
  Demux8/6 -> Subsystem5/6(input5)
  Radians to Degrees4/1 -> Display29/1
  Radians to Degrees5/1 -> Display24/1
  Radians to Degrees8/1 -> Display42/1
  Radians to Degrees7/1 -> Display47/1
  Demux12/6 -> Subsystem11/6(input5)
  Demux12/5 -> Subsystem11/5(input4)
  Demux12/4 -> Subsystem11/4(input3)
  Demux12/3 -> Subsystem11/3(input2)
  Demux12/2 -> Subsystem11/2(input1)
  Demux12/1 -> Subsystem11/1(input0)
  Inverse Kinematics2/2 -> Terminator8/1
  Demux11/1 -> MATLAB Function3/1(theta1)
  Demux10/3 -> Subsystem8/3(input2)
  Mux9/1 -> Subsystem12/1(Radians in)
  Trapezoidal Velocity Profile Trajectory3/2 -> Scope/1
  Trapezoidal Velocity Profile Trajectory2/1 -> Subsystem13/1(In1)
  Trapezoidal Velocity Profile Trajectory3/1 -> Coordinate Transformation Conversion2/1
  Demux11/3 -> MATLAB Function3/3(theta3)
  MATLAB Function3/6(Ry) -> Display40/1
  MATLAB Function3/3(Y) -> XD YD6/2, Display46/1
  Constant5/1 -> Inverse Kinematics2/2
  Coordinate Transformation Conversion2/1 -> Display41/1, Inverse Kinematics2/1
  Constant6/1 -> Inverse Kinematics2/3
  Subsystem8/3(output2) -> Mux8/3
  Demux10/1 -> Subsystem8/1(input0)
  Trapezoidal Velocity Profile Trajectory2/2 -> Terminator12/1
  Radians to Degrees6/1 -> Demux11/1
  Demux10/4 -> Subsystem8/4(input3)
  Subsystem8/1(output) -> Mux8/1
  Demux10/5 -> Subsystem8/5(input4)
  Demux10/2 -> Subsystem8/2(input1)
  Mux8/1 -> Radians to Degrees6/1, Radians to Degrees7/1
  Subsystem8/4(output3) -> Mux8/4
  Subsystem8/2(output1) -> Mux8/2
  Subsystem8/5(output4) -> Mux8/5
  Subsystem8/6(output5) -> Mux8/6
  Demux10/6 -> Subsystem8/6(input5)
  Trapezoidal Velocity Profile Trajectory3/3 -> Terminator10/1
  Trapezoidal Velocity Profile Trajectory2/3 -> Terminator13/1
  Subsystem13/1(Config) -> Demux12/1
  Subsystem13/2(Info) -> Terminator11/1
  MATLAB Function3/5(Rz) -> Display45/1
  Demux11/4 -> MATLAB Function3/4(theta4)
  MATLAB Function3/4(Z) -> Display44/1
  Demux11/5 -> MATLAB Function3/5(theta5)
  MATLAB Function3/1(H) -> Display39/1
  Subsystem11/4(output3) -> Mux9/4
  Subsystem11/2(output1) -> Mux9/2
  Subsystem11/5(output4) -> Mux9/5
  Subsystem11/6(output5) -> Mux9/6
  Subsystem11/1(output) -> Mux9/1
  Subsystem11/3(output2) -> Mux9/3
  Clock4/1 -> Trapezoidal Velocity Profile Trajectory2/1
  Demux11/2 -> MATLAB Function3/2(theta2)
  Demux11/6 -> MATLAB Function3/6(theta6)
  Clock2/1 -> Trapezoidal Velocity Profile Trajectory3/1
  MATLAB Function3/7(Rx) -> Display43/1
  MATLAB Function3/2(X) -> XD YD6/1, Display38/1
  Inverse Kinematics2/1 -> Radians to Degrees8/1, Get Jacobian/1, Demux10/1
  Subsystem8/7(output6) -> Mux10/1
  Subsystem8/8(output7) -> Mux10/2
  Subsystem8/9(output8) -> Mux10/3
  Subsystem8/10(output9) -> Mux10/4
  Subsystem8/11(output10) -> Mux10/5
  Subsystem8/12(output11) -> Mux10/6
  Get Jacobian/1 -> Matrix Multiply/1
  Mux10/1 -> Matrix Multiply/2
  Matrix Multiply/1 -> Demux13/1
  Demux13/1 -> Terminator14/1
  Demux13/2 -> Scope/2
  Radians to Degrees2/1 -> Scope1/2, Demux5/1
  Polynomial Trajectory/1 -> Selector/1, Selector1/1, Gain/1, Scope1/3, Coordinate Transformation Conversion1/1
  Selector/1 -> XY input/1
  Selector1/1 -> XY input/2
  Selector2/1 -> XY out/1
  Selector3/1 -> XY out/2
  Gain/1 -> Display21/1
  MATLAB Function2/2(q) -> Gain1/1, Display17/1, Selector3/1, Selector2/1
  Gain1/1 -> Scope1/4
  Inverse Kinematics3/2 -> Terminator2/1
  Constant4/1 -> Inverse Kinematics3/2
  Coordinate Transformation Conversion3/1 -> Display23/1, Inverse Kinematics3/1
  Constant7/1 -> Inverse Kinematics3/3
  Inverse Kinematics3/1 -> Radians to Degrees3/1
  Clock5/1 -> Polynomial Trajectory14/1
  Polynomial Trajectory14/2 -> Display28/1
  Polynomial Trajectory14/3 -> Display30/1
  Polynomial Trajectory14/1 -> Selector16/1, Selector17/1, Coordinate Transformation Conversion3/1, Display26/1
  Selector4/1 -> Scope2/1
  Selector5/1 -> Scope2/2
  Selector9/1 -> Scope2/6
  Selector8/1 -> Scope2/5
  Selector7/1 -> Scope2/4
  Selector6/1 -> Scope2/3
  Clock7/1 -> Polynomial Trajectory4/1
  Polynomial Trajectory4/2 -> Display48/1
  Polynomial Trajectory4/3 -> Display49/1
  Polynomial Trajectory5/3 -> Display33/1
  Polynomial Trajectory5/2 -> Display32/1
  Polynomial Trajectory5/1 -> Scope5/3, Display31/1
  Clock6/1 -> Polynomial Trajectory5/1
  Clock8/1 -> Polynomial Trajectory6/1
  Polynomial Trajectory6/2 -> Display51/1
  Polynomial Trajectory6/3 -> Display52/1
  Polynomial Trajectory6/1 -> Scope5/2, Display50/1
  Clock9/1 -> MATLAB Function/2(stopFlag)
  Signal Builder2/1(x) -> Display14/1, XY Graph/1, Mux2/1
  Signal Builder4/2(y) -> Display59/1, xy without interpolation2/2, Mux11/2
  Signal Builder4/1(x) -> Display57/1, xy without interpolation2/1, Mux11/1
  Constant9/1 -> Inverse Kinematics4/3
  Signal Builder4/3(z) -> Display58/1, Mux11/3
  Coordinate Transformation Conversion4/1 -> Display56/1, Inverse Kinematics4/1
  Mux11/1 -> Coordinate Transformation Conversion4/1
  Inverse Kinematics4/2 -> Terminator3/1
  Constant8/1 -> Inverse Kinematics4/2
  Clock10/1 -> MATLAB Function4/2(stopFlag)
  Selector12/1 -> Scope6/3
  Selector13/1 -> Scope6/4
  Selector14/1 -> Scope6/5
  Selector15/1 -> Scope6/6
  Selector11/1 -> Scope6/2
  Selector10/1 -> Scope6/1
  Inverse Kinematics4/1 -> Display66/1, Radians to Degrees9/1
  Selector16/1 -> xy with interpolation/1
  Selector17/1 -> xy with interpolation/2
  Polynomial Trajectory7/3 -> Display60/1
  Polynomial Trajectory7/2 -> Display55/1
  Clock11/1 -> Polynomial Trajectory7/1
  Demux6/2 -> MATLAB Function7/2(theta2)
  Demux6/6 -> MATLAB Function7/6(theta6)
  Demux6/1 -> MATLAB Function7/1(theta1)
  Demux6/5 -> MATLAB Function7/5(theta5)
  Demux6/4 -> MATLAB Function7/4(theta4)
  Demux6/3 -> MATLAB Function7/3(theta3)
  Selector18/1 -> xy  interpolation1/1
  Selector19/1 -> xy  interpolation1/2
  MATLAB Function7/2(q) -> Display65/1, Gain3/1, Gain2/1
  MATLAB Function7/3(Rz) -> Display61/1
  MATLAB Function7/4(Ry) -> Display64/1
  MATLAB Function7/5(Rx) -> Display62/1
  MATLAB Function7/1(H) -> Display63/1
  Polynomial Trajectory7/1 -> Scope3/2, Demux6/1, Selector25/1, Selector24/1, Selector23/1, Selector22/1, Selector21/1, Selector20/1, Display54/1
  Selector20/1 -> Scope9/1
  Selector21/1 -> Scope9/2
  Selector25/1 -> Scope9/6
  Selector24/1 -> Scope9/5
  Selector23/1 -> Scope9/4
  Selector22/1 -> Scope9/3
  Gain2/1 -> Selector18/1
  Gain3/1 -> Selector19/1
  Gain5/1 -> Selector27/1
  Gain4/1 -> Selector26/1
  Radians to Degrees3/1 -> Demux7/1, Scope8/1, MATLAB Function/1(q), Display22/1, Selector9/1, Selector8/1, Selector7/1, Selector6/1, Selector5/1, Selector4/1
  MATLAB Function8/1(H) -> Display69/1
  MATLAB Function8/5(Rx) -> Display68/1
  MATLAB Function8/4(Ry) -> Display70/1
  MATLAB Function8/3(Rz) -> Display67/1
  MATLAB Function8/2(q) -> Gain4/1, Gain5/1, Display71/1
  Selector27/1 -> xy  interpolation2/2
  Selector26/1 -> xy  interpolation2/1
  Demux7/3 -> MATLAB Function8/3(theta3)
  Demux7/4 -> MATLAB Function8/4(theta4)
  Demux7/5 -> MATLAB Function8/5(theta5)
  Demux7/1 -> MATLAB Function8/1(theta1)
  Demux7/6 -> MATLAB Function8/6(theta6)
  Demux7/2 -> MATLAB Function8/2(theta2)
  Signal Builder3/1(x) -> xy without interpolation1/1
  Signal Builder3/2(y) -> xy without interpolation1/2
  Signal Builder3/3(z) -> Terminator9/1
  MATLAB Function9/1(H) -> Display74/1
  MATLAB Function9/3(Rz) -> Display72/1
  Selector29/1 -> Scope13/2, xy  interpolation3/2
  Selector28/1 -> Scope13/1, xy  interpolation5/1, xy  interpolation3/1
  Demux14/3 -> MATLAB Function9/3(theta3)
  Demux14/4 -> MATLAB Function9/4(theta4)
  Demux14/5 -> MATLAB Function9/5(theta5)
  Demux14/1 -> MATLAB Function9/1(theta1)
  Demux14/6 -> MATLAB Function9/6(theta6)
  Demux14/2 -> MATLAB Function9/2(theta2)
  Subsystem/1(output) -> Mux13/1
  Subsystem/2(output1) -> Mux13/2
  Demux15/3 -> Subsystem/3(input2)
  Subsystem/6(output5) -> Mux13/6
  Subsystem/4(output3) -> Mux13/4
  Demux15/5 -> Subsystem/5(input4)
  Subsystem/3(output2) -> Mux13/3
  Subsystem/5(output4) -> Mux13/5
  Degrees to Radians1/1 -> Demux15/1
  Mux13/1 -> Radians to Degrees10/1, Display84/1
  Demux15/4 -> Subsystem/4(input3)
  Demux15/2 -> Subsystem/2(input1)
  Demux15/1 -> Subsystem/1(input0)
  Demux15/6 -> Subsystem/6(input5)
  From Workspace5/1 -> Mux14/6
  From Workspace3/1 -> Mux14/4
  From Workspace4/1 -> Mux14/5
  From Workspace1/1 -> Mux14/2
  From Workspace2/1 -> Mux14/3
  From Workspace/1 -> Mux14/1
  Demux17/2 -> MATLAB Function11/2(theta2)
  Demux17/6 -> MATLAB Function11/6(theta6)
  Demux17/1 -> MATLAB Function11/1(theta1)
  Demux17/5 -> MATLAB Function11/5(theta5)
  Demux17/4 -> MATLAB Function11/4(theta4)
  Demux17/3 -> MATLAB Function11/3(theta3)
  Selector30/1 -> xy  interpolation4/1
  Selector31/1 -> xy  interpolation4/2
  MATLAB Function11/2(q) -> Display89/1, Gain9/1, Gain8/1
  MATLAB Function11/3(Rz) -> Display85/1
  MATLAB Function11/4(Ry) -> Display88/1
  MATLAB Function11/5(Rx) -> Display86/1
  MATLAB Function11/1(H) -> Display87/1
  Gain8/1 -> Selector30/1
  Gain9/1 -> Selector31/1
  Radians to Degrees9/1 -> Scope3/1, Display53/1, MATLAB Function4/1(q), Scope10/1, Selector10/1, Selector11/1, Selector12/1, Selector13/1, Selector14/1, Selector15/1
  Polynomial Trajectory10/3 -> Display98/1
  Polynomial Trajectory8/3 -> Display95/1
  Clock14/1 -> Polynomial Trajectory10/1
  Clock12/1 -> Polynomial Trajectory9/1
  Polynomial Trajectory10/1 -> Scope10/2, Display96/1
  Polynomial Trajectory9/2 -> Display91/1
  Polynomial Trajectory9/3 -> Display92/1
  Clock13/1 -> Polynomial Trajectory8/1
  Polynomial Trajectory10/2 -> Display97/1
  Polynomial Trajectory9/1 -> Scope10/3, Display90/1
  Polynomial Trajectory8/2 -> Display94/1
  Polynomial Trajectory8/1 -> Scope11/1, Selector37/1, Selector36/1, Selector35/1, Selector34/1, Selector33/1, Selector32/1, Scope10/4, Display93/1
  Selector32/1 -> Scope12/1
  Selector33/1 -> Scope12/2
  Selector37/1 -> Scope12/6
  Selector36/1 -> Scope12/5
  Selector35/1 -> Scope12/4
  Selector34/1 -> Scope12/3
  Signal Builder5/1(Signal 1) -> Mux4/1
  Signal Builder5/2(Signal 2) -> Mux4/2
  Signal Builder5/3(Signal 3) -> Mux4/3
  Signal Builder5/4(Signal 4) -> Mux4/4
  Signal Builder5/5(Signal 5) -> Mux4/5
  Signal Builder5/6(Signal 6) -> Mux4/6
  Selector38/1 -> Scope13/3, xy  interpolation5/2
  Mux4/1 -> Demux14/1, Scope5/1
  Polynomial Trajectory4/1 -> Demux17/1, Scope7/1, Scope5/4, Display34/1
  Mux14/1 -> Degrees to Radians1/1
  MATLAB Function9/2(q) -> Selector38/1, Selector28/1, Selector29/1, MATLAB Function13/1(q), Display76/1
  Clock15/1 -> MATLAB Function13/2(stopFlag)
  MATLAB Function10/4(Ry) -> Display80/1
  Gain6/1 -> Selector39/1
  MATLAB Function10/2(q) -> Display81/1, Gain7/1, Gain6/1
  Gain7/1 -> Selector40/1
  MATLAB Function10/5(Rx) -> Display78/1
  Demux16/6 -> MATLAB Function10/6(theta6)
  MATLAB Function10/3(Rz) -> Display77/1
  Selector39/1 -> xy  interpolation6/1
  MATLAB Function10/1(H) -> Display79/1
  Demux16/4 -> MATLAB Function10/4(theta4)
  Demux16/5 -> MATLAB Function10/5(theta5)
  Demux16/3 -> MATLAB Function10/3(theta3)
  Demux16/1 -> MATLAB Function10/1(theta1)
  Demux16/2 -> MATLAB Function10/2(theta2)
  Selector40/1 -> xy  interpolation6/2
  Radians to Degrees10/1 -> Demux16/1
  MATLAB Function9/5(Rx) -> Display73/1
  Mux12/1 -> Scope15/1, Degrees to Radians2/1
  Signal Builder11/6(Signal 6) -> Mux12/6
  Signal Builder11/5(Signal 5) -> Mux12/5
  Signal Builder11/4(Signal 4) -> Mux12/4
  Signal Builder11/3(Signal 3) -> Mux12/3
  Signal Builder11/2(Signal 2) -> Mux12/2
  Signal Builder11/1(Signal 1) -> Mux12/1
  Polynomial Trajectory13/1 -> Display103/1, Scope15/2
  Polynomial Trajectory13/3 -> Display105/1
  Polynomial Trajectory13/2 -> Display104/1
  Clock19/1 -> Polynomial Trajectory13/1
  Clock17/1 -> Polynomial Trajectory12/1
  Polynomial Trajectory12/1 -> Display82/1, Scope15/3
  Polynomial Trajectory12/2 -> Display83/1
  Polynomial Trajectory12/3 -> Display99/1
  Polynomial Trajectory11/3 -> Display102/1
  Polynomial Trajectory11/2 -> Display101/1
  Clock18/1 -> Polynomial Trajectory11/1
  Demux18/6 -> Subsystem14/6(input5)
  Demux18/1 -> Subsystem14/1(input0)
  Demux18/2 -> Subsystem14/2(input1)
  Subsystem14/6(output5) -> Mux15/6
  Demux18/3 -> Subsystem14/3(input2)
  Degrees to Radians2/1 -> Radians to Degrees11/1, Demux18/1
  Subsystem14/5(output4) -> Mux15/5
  Subsystem14/3(output2) -> Mux15/3
  Subsystem14/4(output3) -> Mux15/4
  Demux18/5 -> Subsystem14/5(input4)
  Subsystem14/1(output) -> Mux15/1
  Subsystem14/2(output1) -> Mux15/2
  Demux18/4 -> Subsystem14/4(input3)
  Clock16/1 -> MATLAB Function14/2(stopFlag)
  Radians to Degrees11/1 -> MATLAB Function14/1(q)
  Clock20/1 -> MATLAB Function15/2(stopFlag)
  Polynomial Trajectory11/1 -> Display100/1, MATLAB Function15/1(q), Scope15/4, Scope16/1
  MATLAB Function9/4(Ry) -> Display75/1
  Radians to Degrees12/1 -> Display9/1
  Clock21/1 -> Polynomial Trajectory15/1
  Polynomial Trajectory15/2 -> Display108/1
  Polynomial Trajectory15/3 -> Display109/1
  Polynomial Trajectory15/1 -> MATLAB Function12/1(q), Scope14/2, Display107/1
  Clock22/1 -> MATLAB Function12/2(stopFlag)
  Signal Builder15/1(Signal 1) -> Scope14/1
  Constant11/1 -> MATLAB Function16/1(joint1_angles)
  MATLAB Function16/1(q) -> Scope14/3
  Clock23/1 -> MATLAB Function16/2(time_now)
  Clock24/1 -> MATLAB Function17/2(time_now)
  Constant12/1 -> MATLAB Function17/1(joint1_angles)
  MATLAB Function17/1(q) -> Scope14/4
